simulink model "DAQ"  (R2014a)
settings: Solver=FixedStepDiscrete  StartTime=0.0  StopTime=inf  FixedStep=sample_time  RelTol=1e-3
values from neighbouring files (symbols this model uses):
  A_lpf_velocity = 1 + B1_lpf_velocity + B2_lpf_velocity    [daq_params.m]
  B1_lpf_velocity = -2*exp(-lpf_damping*fcut_velocity*sample_time)*cos(fcut_velocity*sample_time*sqrt(1-lpf_damping^2))    [daq_params.m]
  B2_lpf_velocity = exp(-2*lpf_damping*fcut_velocity*sample_time)    [daq_params.m]
  BOOM_MAX_ENCODER_TICKS = 2^17 - 1    (= 131071)    [daq_params.m]
  BOOM_PITCH_CAL_VALUE_RAD = 0    [daq_params.m]
  BOOM_PITCH_CAL_VALUE_TICKS = 63515    [daq_params.m]
  BOOM_PITCH_ENCODER_RAD_PER_TICK = 2*pi / (2^17 * 2)    (= 2.39684498107e-05)    [daq_params.m]
  BOOM_ROLL_CAL_VALUE_RAD = 6*pi/180    (= 0.10471975512)    [daq_params.m]
  BOOM_ROLL_CAL_VALUE_TICKS = 68304    [daq_params.m]
  BOOM_ROLL_ENCODER_RAD_PER_TICK = 2*pi / (2^17 * 7)    (= 6.84812851735e-06)    [daq_params.m]
  BOOM_YAW_ENCODER_RAD_PER_TICK = 2*pi / (2^17 * 9.6)    (= 4.9934270439e-06)    [daq_params.m]
  fcut_smooth = 16*(2*pi)    (= 100.530964915)    [daq_params.m]
  fcut_unwrap = 8*(2*pi)    (= 50.2654824574)    [daq_params.m]
  HIP_ABS_ENCODER_RAD_PER_TICK = 2*pi / 2^13    (= 0.000766990393943)    [daq_params.m]
  HIP_ABS_MAX_ENCODER_TICKS = 2^13 - 1    (= 8191)    [daq_params.m]
  HIP_INC_ENCODER_RAD_PER_TICK = 2*pi / (2500 * 4 * 57)    (= 1.10231321179e-05)    [daq_params.m]
  HIP_INC_MAX_ENCODER_TICKS = 2^16 - 1    (= 65535)    [daq_params.m]
  HIP_MOTOR_CONSTANT = 0.184    [daq_params.m]
  HIP_MTR_GEAR_RATIO = 57    [daq_params.m]
  HIP_MTR_MAX_TORQUE = MTR_HIP_MAX_CURRENT*HIP_MOTOR_CONSTANT*HIP_MTR_GEAR_RATIO    (= 629.28)    [daq_params.m]
  LEFT_HIP_CALIB_POS = 3*pi/2    (= 4.71238898038)    [daq_params.m]
  LEFT_HIP_CALIB_VAL = 1359    [daq_params.m]
  LEFT_MOTOR_HIP_DIRECTION = 1.0    (= 1)    [daq_params.m]
  LEG1_LEG_A_CALIB_VAL = 227806296+18240-105494    (= 227719042)    [daq_params.m]
  LEG1_LEG_A_RAD_PER_CNT = 9.8039216e-09    [daq_params.m]
  LEG1_LEG_B_CALIB_VAL = 227981518-27550+100498    (= 228054466)    [daq_params.m]
  LEG1_LEG_B_RAD_PER_CNT = -9.8039216e-09    [daq_params.m]
  LEG1_MOTOR_A_DIRECTION = 1.0    (= 1)    [daq_params.m]
  LEG1_MOTOR_B_DIRECTION = -1.0    (= -1)    [daq_params.m]
  LEG1_TRAN_A_CALIB_VAL = 162551054    [daq_params.m]
  LEG1_TRAN_A_RAD_PER_CNT = 9.8039216e-09    [daq_params.m]
  LEG1_TRAN_B_CALIB_VAL = 163658926    [daq_params.m]
  LEG1_TRAN_B_RAD_PER_CNT = -9.8039216e-09    [daq_params.m]
  LEG2_LEG_A_CALIB_VAL = 208914429-56335+74466    (= 208932560)    [daq_params.m]
  LEG2_LEG_A_RAD_PER_CNT = -9.8039216e-09    [daq_params.m]
  LEG2_LEG_B_CALIB_VAL = 229010442-9300+102681    (= 229103823)    [daq_params.m]
  LEG2_LEG_B_RAD_PER_CNT = -9.8039216e-09    [daq_params.m]
  LEG2_MOTOR_A_DIRECTION = 1.0    (= 1)    [daq_params.m]
  LEG2_MOTOR_B_DIRECTION = -1.0    (= -1)    [daq_params.m]
  LEG2_TRAN_A_CALIB_VAL = 162423925    [daq_params.m]
  LEG2_TRAN_A_RAD_PER_CNT = 9.8039216e-09    [daq_params.m]
  LEG2_TRAN_B_CALIB_VAL = 177684487    [daq_params.m]
  LEG2_TRAN_B_RAD_PER_CNT = 9.8039216e-09    [daq_params.m]
  LEG_A_CALIB_LOC = 0.959931088596881    (= 0.959931088597)    [daq_params.m]
  LEG_B_CALIB_LOC = 2.181661564992912    (= 2.18166156499)    [daq_params.m]
  LEG_MOTOR_CONSTANT = 0.119    [daq_params.m]
  LEG_MTR_GEAR_RATIO = 50    [daq_params.m]
  LEG_MTR_MAX_TORQUE = MTR_MAX_CURRENT*LEG_MOTOR_CONSTANT*LEG_MTR_GEAR_RATIO    (= 357)    [daq_params.m]
  max_encoder_velocity = 200    [daq_params.m]
  MTR_HIP_MAX_CURRENT = 60.0    (= 60)    [daq_params.m]
  MTR_MAX_COUNT = 19900    [daq_params.m]
  MTR_MAX_CURRENT = 60.0    (= 60)    [daq_params.m]
  RIGHT_HIP_CALIB_POS = -pi/2    (= -1.57079632679)    [daq_params.m]
  RIGHT_HIP_CALIB_VAL = 4444    [daq_params.m]
  RIGHT_MOTOR_HIP_DIRECTION = 1.0    (= 1)    [daq_params.m]
  sensor_start_time = 8    [daq_params.m]
undefined symbols (not defined in the file or in its folder): max_sensor_velocity, sample_time
libraries: xpcethercatlib x158, simulink x15, dspswit3 x1
(part 1 of 3)
settings Model: xpc_rtwmakecfg_data=_xpcethercatlib_  BufferReuse=off  Creator=wmartin  LastModifiedBy=wmartin
settings SolverCC: EnableConcurrentExecution=on
settings DataIOCC: MaxDataPoints=1000000000  SaveFormat=StructureWithTime  SaveOutput=off  SaveTime=off
settings OptimizationCC: BlockReduction=off  OptimizeBlockIOStorage=off  BufferReuse=off  GlobalBufferReuse=off  ExpressionFolding=off  ExpressionDepthLimit=2147483647  LocalBlockOutputs=off  SimCompilerOptimization=On
settings DebuggingCC: UnderspecifiedInitializationDetection=Classic  StateNameClashWarn=warning
settings HardwareCC: ProdIntDivRoundTo=Zero  ProdEndianess=LittleEndian  ProdHWDeviceType=Generic->32-bit x86 compatible
settings ModelReferenceCC: ModelReferenceNumInstancesAllowed=Single  ModelReferenceMinAlgLoopOccurrences=on
settings RTWCC: SystemTargetFile=slrt.tlc  TemplateMakefile=slrt_default_tmf  Description=Simulink Real-Time  RTWVerbose=off  ProcessScript=slrt_make_rtw_hook  RTWCompilerOptimization=On
settings SimulinkRealTimeCC: GeneratePreprocessorConditionals=Disable all  EnableShiftOperators=on  RL32LogBufSizeModifier=100000000

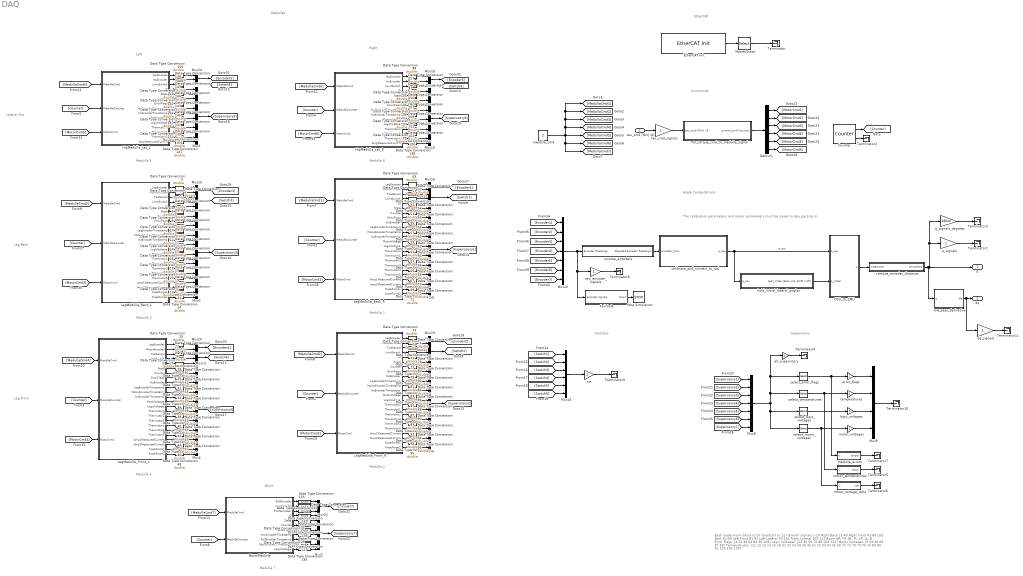
== system DAQ ==
  note: Left
  note: The calibration parameters and motor parameters
      | must be saved in daq_params.m
  note: Right
  note: Lateral Hip
  note: Leg Back
  note: Leg Front
  note: Boom
  note: Medullas
  note: EtherCAT
  note: Angle Computations
  note: Commands
  note: Switches
  note: Supervisory
  note: Medulla 1
  note: Medulla 2
  note: Medulla 4
  note: Medulla 3
  note: Medulla 5
  note: Medulla 6
  note: Medulla 7
  note: Each Supervisory block is 20 (sagittal) or 12 (lateral) signals
      | 1-20      Right Back
      | 21-40     Right Front
      | 41-60     Left Back
      | 61-80     Left Front
      | 81-92     Left Lateral
      | 93-104    Right Lateral
      | 105-112   Boom
      |
      | BR, FR, BL, FL, LR, LL, B
      | Error Flags: [4 24 44 64 84 96 108]
      | Logic Voltages: [10 30 50 70 88 100 112]
      | Motor Voltages: [9 29 49 69 87 99]
      | Temperatures: [11 12 13 14 15 16 31 32 33 34 35 36 51 52 53 54 55 56 71 72 73 74 75 76 89 90 91 101 102 103]
  tau_cmd [Nm] x6 : Inport  OutDataTypeStr=double  PortDimensions=6  SampleTime=0
  BoomMedulla : Subsystem
  Counter : dspswit3/Counter  Direction=Up  CountEvent=Free running  CounterSize=User defined  MaxCount=65535  InitialCount=0  Output=Count and Hit  HitValue=32  ResetInput=off  SamplesPerFrame=1  Ts=.001  CntDtype=double  HitDtype=Logical
  Data Type Conversion{1..111,127..151,157} (137 alike) : DataTypeConversion  OutDataTypeStr=double
  Demux1 : Demux  Outputs=6
  EtherCAT Init : xpcethercatlib/EtherCAT Init   Priority=0  config_file=C:\Users\wmartin\Dropbox\research\atrias\atrias-controller\00 Global Files\atrias_boom.xml  device_id=0  pci_bus=2  pci_slot=2  enaDebug=off  enaDC=on  errLink=off  masterDbg=off  stateChgDbg=off  baseClock=off  masterCfg=off  logFile='E:\dbglog.txt'  sample_time=0.001000
  Fail Safe : Subsystem
  HipMedulla_Lat_L : Subsystem
  HipMedulla_Lat_R : Subsystem
  LegMedulla_Back_L : Subsystem
  LegMedulla_Back_R : Subsystem
  LegMedulla_Front_L : Subsystem
  LegMedulla_Front_R : Subsystem
  MasterState : Selector  InputPortWidth=6  Indices=[2]
  Mux1 : Mux  Inputs=12
  Mux10 : Mux  Inputs=12
  Mux{2,11..13,15..16,18..20,24} (10 alike) : Mux  Inputs=2
  Mux14 : Mux  Inputs=6
  Mux21 : Mux  Inputs=3
  Mux22 : Mux  Inputs=7
  Mux{3..6} (4 alike) : Mux  Inputs=20
  Mux7 : Mux  Inputs=8
  Mux8 : Mux  Inputs=7
  Mux9 : Mux
  OSU_to_CMU : Subsystem
  Stop Simulation : Stop
  Terminator{,1..11} (12 alike) : Terminator
  all_supervisory : Gain
  calibrate_and_convert_to_rad : Subsystem
  dq_signals : Gain
  error_flags : Gain
  hold_initial_lateral_angles : Subsystem
  logic_voltages : Gain
  low_pass_derivative : Subsystem
  medulla_cmd : Constant  Value=2
  medulla_errors : MATLAB Function  TreatAsAtomicUnit=on
  motor_temperatures : MATLAB Function  TreatAsAtomicUnit=on
  motor_voltage_volts : MATLAB Function  TreatAsAtomicUnit=on
  motor_voltages : Gain
  mtr_torque_cmd_to_medulla_signal : Subsystem
  q_signals : Gain
  q_signals_degrees : Gain  Gain=180/pi
  raw_encoder_signals : Gain
  remove_encoder_dropouts : Subsystem
  select_error_flags : Selector  InputPortWidth=112  Indices=[4 24 44 64 84 96 108]
  select_logic_voltages : Selector  InputPortWidth=112  Indices=[10 30 50 70 88 100 112]
  select_motor_voltages : Selector  InputPortWidth=112  Indices=[9 29 49 69 87 99]
  select_temperatures : Selector  InputPortWidth=112  Indices=[11 12 13 14 15 16 31 32 33 34 35 36 51 52 53 54 55 56 71 72 73 74 75 76 89 90 91 101 102 103]
  sw : Gain
  tau_cmd_signals : Gain
  temperatures : Gain
  unwrap_encoders : Subsystem
  q : Outport  OutDataTypeStr=double  PortDimensions=13  SampleTime=[0.001,0]
  dq : Outport  Port=2  OutDataTypeStr=double  PortDimensions=13  SampleTime=[0.001,0]
  wires:
  BoomMedulla/11(LogicVoltage) -> Data Type Conversion136/1
  BoomMedulla/10(PitchEncoderTimestamp) -> Data Type Conversion137/1
  BoomMedulla/9(RollEncoderTimestamp) -> Data Type Conversion127/1
  BoomMedulla/8(YawEncoderTimestamp) -> Data Type Conversion129/1
  BoomMedulla/7(ErrorFlags) -> Data Type Conversion130/1
  BoomMedulla/6(Counter) -> Data Type Conversion128/1
  BoomMedulla/5(State) -> Data Type Conversion134/1
  BoomMedulla/4(ID) -> Data Type Conversion135/1
  BoomMedulla/3(PitchEncoder) -> Data Type Conversion131/1
  BoomMedulla/2(YawEncoder) -> Data Type Conversion132/1
  BoomMedulla/1(RollEncoder) -> Data Type Conversion133/1
  Data Type Conversion133/1 -> Mux21/1
  Data Type Conversion132/1 -> Mux21/2
  Data Type Conversion131/1 -> Mux21/3
  Data Type Conversion135/1 -> Mux7/1
  Data Type Conversion134/1 -> Mux7/2
  Data Type Conversion128/1 -> Mux7/3
  Data Type Conversion130/1 -> Mux7/4
  Data Type Conversion129/1 -> Mux7/5
  Data Type Conversion127/1 -> Mux7/6
  Data Type Conversion137/1 -> Mux7/7
  Data Type Conversion136/1 -> Mux7/8
  HipMedulla_Lat_R/15(AmpMeasuredCurrent) -> Data Type Conversion138/1
  HipMedulla_Lat_R/14(Thermistor2) -> Data Type Conversion99/1
  HipMedulla_Lat_R/13(Thermistor1) -> Data Type Conversion100/1
  HipMedulla_Lat_R/12(Thermistor0) -> Data Type Conversion102/1
  HipMedulla_Lat_R/11(LogicVoltage) -> Data Type Conversion103/1
  HipMedulla_Lat_R/10(MotorVoltage) -> Data Type Conversion101/1
  HipMedulla_Lat_R/9(IncEncoderTimestamp) -> Data Type Conversion108/1
  HipMedulla_Lat_R/8(HipEncoderTimestamp) -> Data Type Conversion109/1
  HipMedulla_Lat_R/7(ErrorFlags) -> Data Type Conversion106/1
  HipMedulla_Lat_R/6(Counter) -> Data Type Conversion107/1
  HipMedulla_Lat_R/5(State) -> Data Type Conversion105/1
  HipMedulla_Lat_R/4(ID) -> Data Type Conversion110/1
  HipMedulla_Lat_R/3(LimitSwitch) -> Data Type Conversion157/1
  HipMedulla_Lat_R/2(IncEncoder) -> Data Type Conversion97/1
  HipMedulla_Lat_R/1(HipEncoder) -> Data Type Conversion98/1
  Data Type Conversion98/1 -> Mux18/1
  Data Type Conversion97/1 -> Mux18/2
  Data Type Conversion110/1 -> Mux10/1
  Data Type Conversion105/1 -> Mux10/2
  Data Type Conversion107/1 -> Mux10/3
  Data Type Conversion106/1 -> Mux10/4
  Data Type Conversion109/1 -> Mux10/5
  Data Type Conversion108/1 -> Mux10/6
  Data Type Conversion101/1 -> Mux10/7
  Data Type Conversion103/1 -> Mux10/8
  Data Type Conversion102/1 -> Mux10/9
  Data Type Conversion100/1 -> Mux10/10
  Data Type Conversion99/1 -> Mux10/11
  mtr_torque_cmd_to_medulla_signal/1(current_cmd [counts]) -> Demux1/1
  Data Type Conversion50/1 -> Mux16/2
  Data Type Conversion49/1 -> Mux16/1
  Data Type Conversion48/1 -> Mux4/20
  Data Type Conversion47/1 -> Mux4/19
  Data Type Conversion46/1 -> Mux4/18
  Data Type Conversion45/1 -> Mux4/17
  Data Type Conversion44/1 -> Mux4/16
  Data Type Conversion43/1 -> Mux4/15
  Data Type Conversion42/1 -> Mux4/14
  Data Type Conversion41/1 -> Mux4/13
  Data Type Conversion40/1 -> Mux4/12
  Data Type Conversion39/1 -> Mux4/11
  Data Type Conversion38/1 -> Mux4/10
  Data Type Conversion37/1 -> Mux4/9
  Data Type Conversion36/1 -> Mux4/8
  Data Type Conversion35/1 -> Mux4/7
  Data Type Conversion34/1 -> Mux4/6
  Data Type Conversion33/1 -> Mux4/5
  Data Type Conversion32/1 -> Mux4/4
  Data Type Conversion31/1 -> Mux4/3
  Data Type Conversion30/1 -> Mux4/2
  Data Type Conversion29/1 -> Mux4/1
  Data Type Conversion28/1 -> Mux13/2
  Data Type Conversion27/1 -> Mux13/1
  Data Type Conversion26/1 -> Mux20/2
  Data Type Conversion25/1 -> Mux20/1
  Data Type Conversion24/1 -> Mux3/20
  Data Type Conversion23/1 -> Mux3/19
  Data Type Conversion22/1 -> Mux3/18
  Data Type Conversion21/1 -> Mux3/17
  Data Type Conversion20/1 -> Mux3/16
  Data Type Conversion19/1 -> Mux3/15
  Data Type Conversion18/1 -> Mux3/14
  Data Type Conversion17/1 -> Mux3/13
  Data Type Conversion16/1 -> Mux3/12
  Data Type Conversion15/1 -> Mux3/11
  Data Type Conversion14/1 -> Mux3/10
  Data Type Conversion13/1 -> Mux3/9
  Data Type Conversion12/1 -> Mux3/8
  Data Type Conversion11/1 -> Mux3/7
  Data Type Conversion10/1 -> Mux3/6
  Data Type Conversion9/1 -> Mux3/5
  Data Type Conversion8/1 -> Mux3/4
  Data Type Conversion7/1 -> Mux3/3
  Data Type Conversion6/1 -> Mux3/2
  Data Type Conversion5/1 -> Mux3/1
  Data Type Conversion4/1 -> Mux2/2
  Data Type Conversion2/1 -> Mux2/1
  Data Type Conversion1/1 -> Mux15/2
  Data Type Conversion3/1 -> Mux15/1
  LegMedulla_Back_R/1(LegEncoder) -> Data Type Conversion49/1
  LegMedulla_Back_L/1(LegEncoder) -> Data Type Conversion3/1
  LegMedulla_Back_R/2(MotorEncoder) -> Data Type Conversion50/1
  tau_cmd [Nm] x6/1 -> tau_cmd_signals/1
  Data Type Conversion138/1 -> Mux10/12
  Data Type Conversion96/1 -> Mux6/20
  Data Type Conversion95/1 -> Mux6/19
  Data Type Conversion94/1 -> Mux6/18
  Data Type Conversion93/1 -> Mux6/17
  Data Type Conversion92/1 -> Mux6/16
  Data Type Conversion91/1 -> Mux6/15
  Data Type Conversion90/1 -> Mux6/14
  Data Type Conversion89/1 -> Mux6/13
  Data Type Conversion88/1 -> Mux6/12
  Data Type Conversion87/1 -> Mux6/11
  Data Type Conversion86/1 -> Mux6/10
  Data Type Conversion85/1 -> Mux6/9
  Data Type Conversion84/1 -> Mux6/8
  Data Type Conversion83/1 -> Mux6/7
  Data Type Conversion82/1 -> Mux6/6
  Data Type Conversion81/1 -> Mux6/5
  Data Type Conversion80/1 -> Mux6/4
  Data Type Conversion79/1 -> Mux6/3
  Data Type Conversion78/1 -> Mux6/2
  Data Type Conversion77/1 -> Mux6/1
  Data Type Conversion76/1 -> Mux12/2
  Data Type Conversion75/1 -> Mux12/1
  Data Type Conversion74/1 -> Mux19/2
  Data Type Conversion73/1 -> Mux19/1
  Data Type Conversion72/1 -> Mux5/20
  Data Type Conversion71/1 -> Mux5/19
  Data Type Conversion70/1 -> Mux5/18
  Data Type Conversion69/1 -> Mux5/17
  Data Type Conversion68/1 -> Mux5/16
  Data Type Conversion67/1 -> Mux5/15
  Data Type Conversion66/1 -> Mux5/14
  Data Type Conversion65/1 -> Mux5/13
  Data Type Conversion64/1 -> Mux5/12
  Data Type Conversion63/1 -> Mux5/11
  Data Type Conversion62/1 -> Mux5/10
  Data Type Conversion61/1 -> Mux5/9
  Data Type Conversion60/1 -> Mux5/8
  Data Type Conversion59/1 -> Mux5/7
  Data Type Conversion58/1 -> Mux5/6
  Data Type Conversion57/1 -> Mux5/5
  Data Type Conversion56/1 -> Mux5/4
  Data Type Conversion55/1 -> Mux5/3
  Data Type Conversion54/1 -> Mux5/2
  Data Type Conversion53/1 -> Mux5/1
  Data Type Conversion52/1 -> Mux11/2
  Data Type Conversion51/1 -> Mux11/1
  LegMedulla_Front_R/3(ToeSensor) -> Data Type Conversion75/1
  LegMedulla_Front_R/2(MotorEncoder) -> Data Type Conversion74/1
  LegMedulla_Front_R/1(LegEncoder) -> Data Type Conversion73/1
  Counter/2 -> Terminator2/1
  LegMedulla_Front_R/24(KneeForce2) -> Data Type Conversion96/1
  LegMedulla_Back_R/24(KneeForce2) -> Data Type Conversion72/1
  LegMedulla_Front_R/23(KneeForce1) -> Data Type Conversion95/1
  LegMedulla_Front_R/22(Amp2MeasuredCurrent) -> Data Type Conversion94/1
  LegMedulla_Front_R/21(Amp1MeasuredCurrent) -> Data Type Conversion93/1
  LegMedulla_Front_R/20(Thermistor5) -> Data Type Conversion92/1
  LegMedulla_Front_R/19(Thermistor4) -> Data Type Conversion91/1
  LegMedulla_Front_R/18(Thermistor3) -> Data Type Conversion90/1
  LegMedulla_Front_R/17(Thermistor2) -> Data Type Conversion89/1
  LegMedulla_Front_R/16(Thermistor1) -> Data Type Conversion88/1
  LegMedulla_Front_R/15(Thermistor0) -> Data Type Conversion87/1
  LegMedulla_Front_R/14(LogicVoltage) -> Data Type Conversion86/1
  LegMedulla_Front_R/13(MotorVoltage) -> Data Type Conversion85/1
  LegMedulla_Front_R/12(IncEncoderTimestamp) -> Data Type Conversion84/1
  LegMedulla_Front_R/11(MotorEncoderTimestamp) -> Data Type Conversion83/1
  LegMedulla_Front_R/10(LegEncoderTimestamp) -> Data Type Conversion82/1
  LegMedulla_Front_R/9(IncEncoder) -> Data Type Conversion81/1
  LegMedulla_Front_R/8(ErrorFlags) -> Data Type Conversion80/1
  LegMedulla_Front_R/7(Counter) -> Data Type Conversion79/1
  LegMedulla_Front_R/6(State) -> Data Type Conversion78/1
  LegMedulla_Front_R/5(ID) -> Data Type Conversion77/1
  LegMedulla_Front_R/4(LimitSwitch) -> Data Type Conversion76/1
  LegMedulla_Back_R/23(KneeForce1) -> Data Type Conversion71/1
  LegMedulla_Back_R/22(Amp2MeasuredCurrent) -> Data Type Conversion70/1
  LegMedulla_Back_R/21(Amp1MeasuredCurrent) -> Data Type Conversion69/1
  LegMedulla_Back_R/20(Thermistor5) -> Data Type Conversion68/1
  LegMedulla_Back_R/19(Thermistor4) -> Data Type Conversion67/1
  LegMedulla_Back_R/18(Thermistor3) -> Data Type Conversion66/1
  LegMedulla_Back_R/17(Thermistor2) -> Data Type Conversion65/1
  LegMedulla_Back_R/16(Thermistor1) -> Data Type Conversion64/1
  LegMedulla_Back_R/15(Thermistor0) -> Data Type Conversion63/1
  LegMedulla_Back_R/14(LogicVoltage) -> Data Type Conversion62/1
  LegMedulla_Back_R/13(MotorVoltage) -> Data Type Conversion61/1
  LegMedulla_Back_R/12(IncEncoderTimestamp) -> Data Type Conversion60/1
  LegMedulla_Back_R/11(MotorEncoderTimestamp) -> Data Type Conversion59/1
  LegMedulla_Back_R/10(LegEncoderTimestamp) -> Data Type Conversion58/1
  LegMedulla_Back_R/9(IncEncoder) -> Data Type Conversion57/1
  LegMedulla_Back_R/8(ErrorFlags) -> Data Type Conversion56/1
  LegMedulla_Back_R/7(Counter) -> Data Type Conversion55/1
  LegMedulla_Back_R/6(State) -> Data Type Conversion54/1
  LegMedulla_Back_R/5(ID) -> Data Type Conversion53/1
  LegMedulla_Back_R/4(LimitSwitch) -> Data Type Conversion52/1
  LegMedulla_Back_R/3(ToeSensor) -> Data Type Conversion51/1
  LegMedulla_Front_L/24(KneeForce2) -> Data Type Conversion48/1
  LegMedulla_Back_L/24(KneeForce2) -> Data Type Conversion24/1
  LegMedulla_Front_L/23(KneeForce1) -> Data Type Conversion47/1
  LegMedulla_Front_L/22(Amp2MeasuredCurrent) -> Data Type Conversion46/1
  LegMedulla_Front_L/21(Amp1MeasuredCurrent) -> Data Type Conversion45/1
  LegMedulla_Front_L/20(Thermistor5) -> Data Type Conversion44/1
  LegMedulla_Front_L/19(Thermistor4) -> Data Type Conversion43/1
  LegMedulla_Front_L/18(Thermistor3) -> Data Type Conversion42/1
  LegMedulla_Front_L/17(Thermistor2) -> Data Type Conversion41/1
  LegMedulla_Front_L/16(Thermistor1) -> Data Type Conversion40/1
  LegMedulla_Front_L/15(Thermistor0) -> Data Type Conversion39/1
  LegMedulla_Front_L/14(LogicVoltage) -> Data Type Conversion38/1
  LegMedulla_Front_L/13(MotorVoltage) -> Data Type Conversion37/1
  LegMedulla_Front_L/12(IncEncoderTimestamp) -> Data Type Conversion36/1
  LegMedulla_Front_L/11(MotorEncoderTimestamp) -> Data Type Conversion35/1
  LegMedulla_Front_L/10(LegEncoderTimestamp) -> Data Type Conversion34/1
  LegMedulla_Front_L/9(IncEncoder) -> Data Type Conversion33/1
  LegMedulla_Front_L/8(ErrorFlags) -> Data Type Conversion32/1
  LegMedulla_Front_L/7(Counter) -> Data Type Conversion31/1
  LegMedulla_Front_L/6(State) -> Data Type Conversion30/1
  LegMedulla_Front_L/5(ID) -> Data Type Conversion29/1
  LegMedulla_Front_L/4(LimitSwitch) -> Data Type Conversion28/1
  LegMedulla_Front_L/3(ToeSensor) -> Data Type Conversion27/1
  LegMedulla_Front_L/2(MotorEncoder) -> Data Type Conversion26/1
  LegMedulla_Front_L/1(LegEncoder) -> Data Type Conversion25/1
  LegMedulla_Back_L/23(KneeForce1) -> Data Type Conversion23/1
  LegMedulla_Back_L/22(Amp2MeasuredCurrent) -> Data Type Conversion22/1
  LegMedulla_Back_L/21(Amp1MeasuredCurrent) -> Data Type Conversion21/1
  LegMedulla_Back_L/20(Thermistor5) -> Data Type Conversion20/1
  LegMedulla_Back_L/19(Thermistor4) -> Data Type Conversion19/1
  LegMedulla_Back_L/18(Thermistor3) -> Data Type Conversion18/1
  LegMedulla_Back_L/17(Thermistor2) -> Data Type Conversion17/1
  LegMedulla_Back_L/16(Thermistor1) -> Data Type Conversion16/1
  LegMedulla_Back_L/15(Thermistor0) -> Data Type Conversion15/1
  LegMedulla_Back_L/14(LogicVoltage) -> Data Type Conversion14/1
  LegMedulla_Back_L/13(MotorVoltage) -> Data Type Conversion13/1
  LegMedulla_Back_L/12(IncEncoderTimestamp) -> Data Type Conversion12/1
  LegMedulla_Back_L/11(MotorEncoderTimestamp) -> Data Type Conversion11/1
  LegMedulla_Back_L/10(LegEncoderTimestamp) -> Data Type Conversion10/1
  LegMedulla_Back_L/9(IncEncoder) -> Data Type Conversion9/1
  LegMedulla_Back_L/8(ErrorFlags) -> Data Type Conversion8/1
  LegMedulla_Back_L/7(Counter) -> Data Type Conversion7/1
  LegMedulla_Back_L/6(State) -> Data Type Conversion6/1
  LegMedulla_Back_L/5(ID) -> Data Type Conversion5/1
  LegMedulla_Back_L/4(LimitSwitch) -> Data Type Conversion4/1
  LegMedulla_Back_L/3(ToeSensor) -> Data Type Conversion2/1
  LegMedulla_Back_L/2(MotorEncoder) -> Data Type Conversion1/1
  Counter/1 -> [Counter]
  [Counter] -> LegMedulla_Back_L/2(MedullaCounter)
  [Counter] -> LegMedulla_Front_L/2(MedullaCounter)
  [Counter] -> LegMedulla_Back_R/2(MedullaCounter)
  [Counter] -> LegMedulla_Front_R/2(MedullaCounter)
  [Counter] -> HipMedulla_Lat_R/2(MedullaCounter)
  [Counter] -> HipMedulla_Lat_L/2(MedullaCounter)
  [Counter] -> BoomMedulla/2(MedullaCounter)
  medulla_cmd/1 -> [MedullaCmd7], [MedullaCmd6], [MedullaCmd5], [MedullaCmd4], [MedullaCmd3], [MedullaCmd2], [MedullaCmd1]
  [MedullaCmd3] -> LegMedulla_Back_L/1(MedullaCmd)
  [MedullaCmd4] -> LegMedulla_Front_L/1(MedullaCmd)
  [MedullaCmd1] -> LegMedulla_Back_R/1(MedullaCmd)
  [MedullaCmd2] -> LegMedulla_Front_R/1(MedullaCmd)
  [MedullaCmd6] -> HipMedulla_Lat_R/1(MedullaCmd)
  [MedullaCmd7] -> BoomMedulla/1(MedullaCmd)
  [MedullaCmd5] -> HipMedulla_Lat_L/1(MedullaCmd)
  Data Type Conversion157/1 -> [Switch6]
  [Switch1] -> Mux14/1
  [Switch2] -> Mux14/2
  [Switch3] -> Mux14/3
  [Switch4] -> Mux14/4
  [Switch5] -> Mux14/5
  [Switch6] -> Mux14/6
  low_pass_derivative/1(dq) -> dq_signals/1, dq/1
  calibrate_and_convert_to_rad/1(q_osu) -> OSU_to_CMU/1(q_osu), hold_initial_lateral_angles/1(q_osu)  "q_osu"
  hold_initial_lateral_angles/1(qLat_initial [absL incL absR incR]) -> OSU_to_CMU/2(q_initial)
  [MotorCmd3] -> LegMedulla_Back_L/3(MotorCmd)
  [MotorCmd4] -> LegMedulla_Front_L/3(MotorCmd)
  [MotorCmd1] -> LegMedulla_Back_R/3(MotorCmd)
  [MotorCmd2] -> LegMedulla_Front_R/3(MotorCmd)
  [MotorCmd6] -> HipMedulla_Lat_R/3(MotorCmd)
  [MotorCmd5] -> HipMedulla_Lat_L/3(MotorCmd)
  Demux1/1 -> [MotorCmd1]
  Demux1/2 -> [MotorCmd2]
  Demux1/3 -> [MotorCmd3]
  Demux1/4 -> [MotorCmd4]
  Demux1/5 -> [MotorCmd5]
  Demux1/6 -> [MotorCmd6]
  Mux2/1 -> [Switch3]
  Mux3/1 -> [Supervisory3]
  Mux4/1 -> [Supervisory4]
  Mux5/1 -> [Supervisory1]
  Mux6/1 -> [Supervisory2]
  Mux7/1 -> [Supervisory7]
  [Supervisory1] -> Mux8/1
  [Supervisory2] -> Mux8/2
  [Supervisory3] -> Mux8/3
  [Supervisory4] -> Mux8/4
  [Supervisory5] -> Mux8/5
  [Supervisory6] -> Mux8/6
  [Supervisory7] -> Mux8/7
  Mux10/1 -> [Supervisory6]
  Mux11/1 -> [Switch1]
  Mux12/1 -> [Switch2]
  Mux13/1 -> [Switch4]
  Mux14/1 -> sw/1
  Mux15/1 -> [Encoder3]
  Mux16/1 -> [Encoder1]
  Mux18/1 -> [Encoder6]
  Mux19/1 -> [Encoder2]
  Mux20/1 -> [Encoder4]
  Mux21/1 -> [Encoder7]
  [Encoder7] -> Mux22/7
  [Encoder6] -> Mux22/6
  [Encoder5] -> Mux22/5
  [Encoder4] -> Mux22/4
  [Encoder3] -> Mux22/3
  [Encoder2] -> Mux22/2
  [Encoder1] -> Mux22/1
  Mux22/1 -> unwrap_encoders/1(Encoder Readings), raw_encoder_signals/1, Fail Safe/1(encoder signals)
  HipMedulla_Lat_L/15(AmpMeasuredCurrent) -> Data Type Conversion147/1
  HipMedulla_Lat_L/14(Thermistor2) -> Data Type Conversion151/1
  HipMedulla_Lat_L/13(Thermistor1) -> Data Type Conversion104/1
  HipMedulla_Lat_L/12(Thermistor0) -> Data Type Conversion139/1
  HipMedulla_Lat_L/11(LogicVoltage) -> Data Type Conversion140/1
  HipMedulla_Lat_L/10(MotorVoltage) -> Data Type Conversion111/1
  HipMedulla_Lat_L/9(IncEncoderTimestamp) -> Data Type Conversion144/1
  HipMedulla_Lat_L/8(HipEncoderTimestamp) -> Data Type Conversion145/1
  HipMedulla_Lat_L/7(ErrorFlags) -> Data Type Conversion142/1
  HipMedulla_Lat_L/6(Counter) -> Data Type Conversion143/1
  HipMedulla_Lat_L/5(State) -> Data Type Conversion141/1
  HipMedulla_Lat_L/4(ID) -> Data Type Conversion146/1
  HipMedulla_Lat_L/3(LimitSwitch) -> Data Type Conversion148/1
  HipMedulla_Lat_L/2(IncEncoder) -> Data Type Conversion149/1
  HipMedulla_Lat_L/1(HipEncoder) -> Data Type Conversion150/1
  Data Type Conversion150/1 -> Mux24/1
  Data Type Conversion149/1 -> Mux24/2
  Data Type Conversion146/1 -> Mux1/1
  Data Type Conversion141/1 -> Mux1/2
  Data Type Conversion143/1 -> Mux1/3
  Data Type Conversion142/1 -> Mux1/4
  Data Type Conversion145/1 -> Mux1/5
  Data Type Conversion144/1 -> Mux1/6
  Data Type Conversion111/1 -> Mux1/7
  Data Type Conversion140/1 -> Mux1/8
  Data Type Conversion139/1 -> Mux1/9
  Data Type Conversion104/1 -> Mux1/10
  Data Type Conversion151/1 -> Mux1/11
  Data Type Conversion147/1 -> Mux1/12
  Data Type Conversion148/1 -> [Switch5]
  Mux1/1 -> [Supervisory5]
  Mux24/1 -> [Encoder5]
  q_signals/1 -> Terminator1/1
  tau_cmd_signals/1 -> mtr_torque_cmd_to_medulla_signal/1(tau_cmd [Nm] x6)
  Mux8/1 -> select_temperatures/1, select_error_flags/1, all_supervisory/1, select_motor_voltages/1, select_logic_voltages/1
  select_error_flags/1 -> error_flags/1, medulla_errors/1(u)
  select_temperatures/1 -> temperatures/1, motor_temperatures/1(u)
  select_logic_voltages/1 -> logic_voltages/1
  select_motor_voltages/1 -> motor_voltages/1, motor_voltage_volts/1(u)
  error_flags/1 -> Mux9/1
  temperatures/1 -> Mux9/2
  logic_voltages/1 -> Mux9/3
  motor_voltages/1 -> Mux9/4
  Mux9/1 -> Terminator10/1
  q_signals_degrees/1 -> Terminator3/1
  OSU_to_CMU/1(q) -> remove_encoder_dropouts/1(measured)
  EtherCAT Init/1 -> MasterState/1
  all_supervisory/1 -> Terminator4/1
  motor_temperatures/1(temp) -> Terminator5/1
  motor_voltage_volts/1(volt) -> Terminator6/1
  medulla_errors/1(errors) -> Terminator7/1
  MasterState/1 -> Terminator/1
  raw_encoder_signals/1 -> Terminator8/1
  sw/1 -> Terminator9/1
  remove_encoder_dropouts/1(smoothed) -> low_pass_derivative/1(q), q_signals/1, q_signals_degrees/1, q/1
  unwrap_encoders/1(Adjusted Encoder Readings) -> calibrate_and_convert_to_rad/1(encoder_ticks)
  Fail Safe/1(stop?) -> Stop Simulation/1
  dq_signals/1 -> Terminator11/1

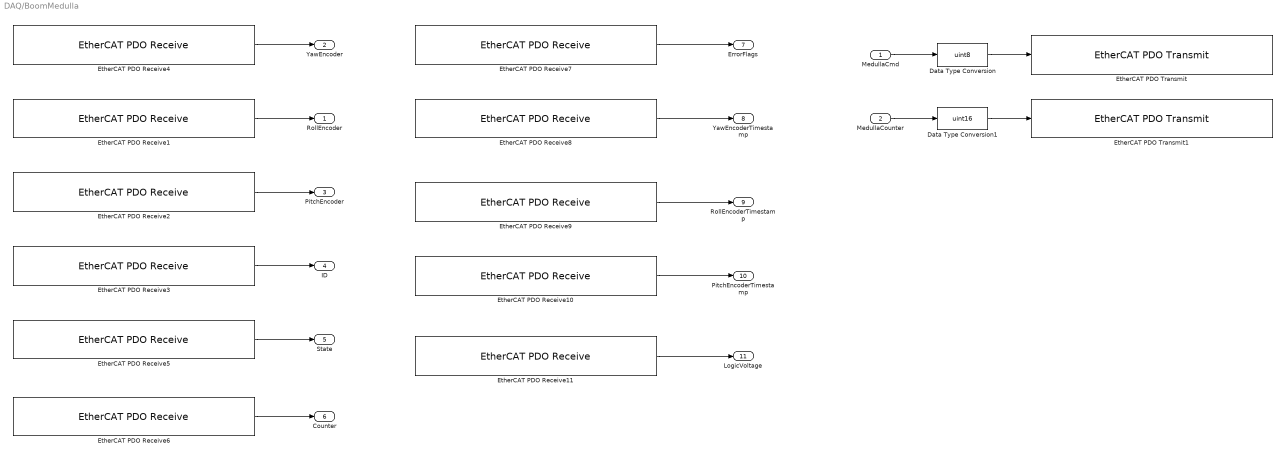
== system DAQ/BoomMedulla ==
  MedullaCmd : Inport
  MedullaCounter : Inport  Port=2
  Data Type Conversion : DataTypeConversion  OutDataTypeStr=uint8
  Data Type Conversion1 : DataTypeConversion  OutDataTypeStr=uint16
  EtherCAT PDO Receive1 : xpcethercatlib/EtherCAT PDO Receive  Priority=2  sig_name=Box 7 (ATRIAS 2.1 Boom (Medulla 1.5)).X Encoder.Encoder  sig_offset=2432  sig_type=uint32  type_size=32  sig_dim=1  device_id=0  sample_time=0.001000
  EtherCAT PDO Receive10 : xpcethercatlib/EtherCAT PDO Receive  Priority=2  sig_name=Box 7 (ATRIAS 2.1 Boom (Medulla 1.5)).Pitch Encoder.Timestamp  sig_offset=2512  sig_type=uint16  type_size=16  sig_dim=1  device_id=0  sample_time=0.001000
  EtherCAT PDO Receive11 : xpcethercatlib/EtherCAT PDO Receive  Priority=2  sig_name=Box 7 (ATRIAS 2.1 Boom (Medulla 1.5)).Power.Logic Voltage  sig_offset=2576  sig_type=uint16  type_size=16  sig_dim=1  device_id=0  sample_time=0.001000
  EtherCAT PDO Receive2 : xpcethercatlib/EtherCAT PDO Receive  Priority=2  sig_name=Box 7 (ATRIAS 2.1 Boom (Medulla 1.5)).Pitch Encoder.Encoder  sig_offset=2480  sig_type=uint32  type_size=32  sig_dim=1  device_id=0  sample_time=0.001000
  EtherCAT PDO Receive3 : xpcethercatlib/EtherCAT PDO Receive  Priority=2  sig_name=Box 7 (ATRIAS 2.1 Boom (Medulla 1.5)).uController Status.ID  sig_offset=2400  sig_type=uint8  type_size=8  sig_dim=1  device_id=0  sample_time=0.001000
  EtherCAT PDO Receive4 : xpcethercatlib/EtherCAT PDO Receive  Priority=2  sig_name=Box 7 (ATRIAS 2.1 Boom (Medulla 1.5)).Z Encoder.Encoder  sig_offset=2528  sig_type=uint32  type_size=32  sig_dim=1  device_id=0  sample_time=0.001000
  EtherCAT PDO Receive5 : xpcethercatlib/EtherCAT PDO Receive  Priority=2  sig_name=Box 7 (ATRIAS 2.1 Boom (Medulla 1.5)).uController Status.State  sig_offset=2408  sig_type=uint8  type_size=8  sig_dim=1  device_id=0  sample_time=0.001000
  EtherCAT PDO Receive6 : xpcethercatlib/EtherCAT PDO Receive  Priority=2  sig_name=Box 7 (ATRIAS 2.1 Boom (Medulla 1.5)).uController Status.Counter  sig_offset=2416  sig_type=uint8  type_size=8  sig_dim=1  device_id=0  sample_time=0.001000
  EtherCAT PDO Receive7 : xpcethercatlib/EtherCAT PDO Receive  Priority=2  sig_name=Box 7 (ATRIAS 2.1 Boom (Medulla 1.5)).uController Status.Error Flags  sig_offset=2424  sig_type=uint8  type_size=8  sig_dim=1  device_id=0  sample_time=0.001000
  EtherCAT PDO Receive8 : xpcethercatlib/EtherCAT PDO Receive  Priority=2  sig_name=Box 7 (ATRIAS 2.1 Boom (Medulla 1.5)).Z Encoder.Timestamp  sig_offset=2560  sig_type=uint16  type_size=16  sig_dim=1  device_id=0  sample_time=0.001000
  EtherCAT PDO Receive9 : xpcethercatlib/EtherCAT PDO Receive  Priority=2  sig_name=Box 7 (ATRIAS 2.1 Boom (Medulla 1.5)).X Encoder.Timestamp  sig_offset=2464  sig_type=uint16  type_size=16  sig_dim=1  device_id=0  sample_time=0.001000
  EtherCAT PDO Transmit : xpcethercatlib/EtherCAT PDO Transmit   Priority=3  sig_name=Box 7 (ATRIAS 2.1 Boom (Medulla 1.5)).uControllerInput.Command  sig_offset=2400  sig_type=uint8  type_size=8  sig_dim=1  device_id=0  sample_time=0.001000
  EtherCAT PDO Transmit1 : xpcethercatlib/EtherCAT PDO Transmit   Priority=3  sig_name=Box 7 (ATRIAS 2.1 Boom (Medulla 1.5)).uControllerInput.Counter  sig_offset=2408  sig_type=uint16  type_size=16  sig_dim=1  device_id=0  sample_time=0.001000
  RollEncoder : Outport
  YawEncoder : Outport  Port=2
  PitchEncoder : Outport  Port=3
  ID : Outport  Port=4
  State : Outport  Port=5
  Counter : Outport  Port=6
  ErrorFlags : Outport  Port=7
  YawEncoderTimestamp : Outport  Port=8
  RollEncoderTimestamp : Outport  Port=9
  PitchEncoderTimestamp : Outport  Port=10
  LogicVoltage : Outport  Port=11
  wires:
  Data Type Conversion/1 -> EtherCAT PDO Transmit/1
  Data Type Conversion1/1 -> EtherCAT PDO Transmit1/1
  MedullaCmd/1 -> Data Type Conversion/1
  MedullaCounter/1 -> Data Type Conversion1/1
  EtherCAT PDO Receive4/1 -> YawEncoder/1
  EtherCAT PDO Receive1/1 -> RollEncoder/1
  EtherCAT PDO Receive2/1 -> PitchEncoder/1
  EtherCAT PDO Receive3/1 -> ID/1
  EtherCAT PDO Receive5/1 -> State/1
  EtherCAT PDO Receive6/1 -> Counter/1
  EtherCAT PDO Receive7/1 -> ErrorFlags/1
  EtherCAT PDO Receive8/1 -> YawEncoderTimestamp/1
  EtherCAT PDO Receive9/1 -> RollEncoderTimestamp/1
  EtherCAT PDO Receive10/1 -> PitchEncoderTimestamp/1
  EtherCAT PDO Receive11/1 -> LogicVoltage/1

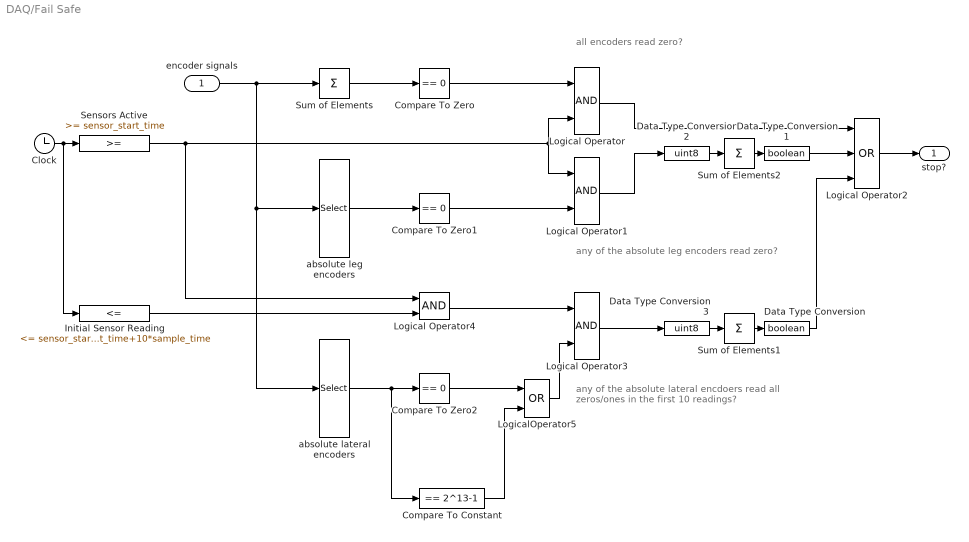
== system DAQ/Fail Safe ==
  note: any of the absolute leg encoders read zero?
  note: all encoders read zero?
  note: any of the absolute lateral encdoers read all
      | zeros/ones in the first 10 readings?
  encoder signals : Inport
  Clock : Clock
  Compare To Constant : simulink/Logic and Bit Operations/Compare To Constant  relop===  const=2^13-1  OutDataTypeStr=boolean
  Compare To Zero : simulink/Logic and Bit Operations/Compare To Zero  relop===  OutDataTypeStr=boolean
  Compare To Zero1 : simulink/Logic and Bit Operations/Compare To Zero  relop===  OutDataTypeStr=boolean
  Compare To Zero2 : simulink/Logic and Bit Operations/Compare To Zero  relop===  OutDataTypeStr=boolean
  Data Type Conversion : DataTypeConversion  OutDataTypeStr=boolean
  Data Type Conversion1 : DataTypeConversion  OutDataTypeStr=boolean
  Data Type Conversion2 : DataTypeConversion  OutDataTypeStr=uint8
  Data Type Conversion3 : DataTypeConversion  OutDataTypeStr=uint8
  Initial Sensor Reading : simulink/Logic and Bit Operations/Compare To Constant  relop=<=  const=sensor_start_time+10*sample_time  OutDataTypeStr=boolean
  Logical Operator{,1,3..4} (4 alike) : Logic  AllPortsSameDT=off  OutDataTypeStr=boolean
  Logical Operator2 : Logic  Operator=OR  Inputs=3  AllPortsSameDT=off  OutDataTypeStr=boolean
  LogicalOperator5 : Logic  Operator=OR  AllPortsSameDT=off  OutDataTypeStr=boolean
  Sensors Active : simulink/Logic and Bit Operations/Compare To Constant  relop=>=  const=sensor_start_time  OutDataTypeStr=boolean
  Sum of Elements : Sum  Inputs=+
  Sum of Elements1 : Sum  Inputs=+
  Sum of Elements2 : Sum  Inputs=+
  absolute lateral encoders : Selector  InputPortWidth=15  Indices=[9 11]
  absolute leg encoders : Selector  InputPortWidth=15  Indices=[1 2 3 4 5 6 7 8]
  stop? : Outport
  wires:
  LogicalOperator5/1 -> Logical Operator3/2
  Compare To Constant/1 -> LogicalOperator5/2
  Compare To Zero2/1 -> LogicalOperator5/1
  absolute leg encoders/1 -> Compare To Zero1/1
  Compare To Zero1/1 -> Logical Operator1/2
  Logical Operator2/1 -> stop?/1
  Logical Operator1/1 -> Data Type Conversion2/1
  Compare To Zero/1 -> Logical Operator/1
  encoder signals/1 -> absolute lateral encoders/1, absolute leg encoders/1, Sum of Elements/1
  Logical Operator/1 -> Logical Operator2/1
  Sum of Elements/1 -> Compare To Zero/1
  Sensors Active/1 -> Logical Operator4/1, Logical Operator/2, Logical Operator1/1
  absolute lateral encoders/1 -> Compare To Zero2/1, Compare To Constant/1
  Clock/1 -> Initial Sensor Reading/1, Sensors Active/1
  Initial Sensor Reading/1 -> Logical Operator4/2
  Logical Operator4/1 -> Logical Operator3/1
  Logical Operator3/1 -> Data Type Conversion3/1
  Sum of Elements1/1 -> Data Type Conversion/1
  Sum of Elements2/1 -> Data Type Conversion1/1
  Data Type Conversion/1 -> Logical Operator2/3
  Data Type Conversion1/1 -> Logical Operator2/2
  Data Type Conversion2/1 -> Sum of Elements2/1
  Data Type Conversion3/1 -> Sum of Elements1/1

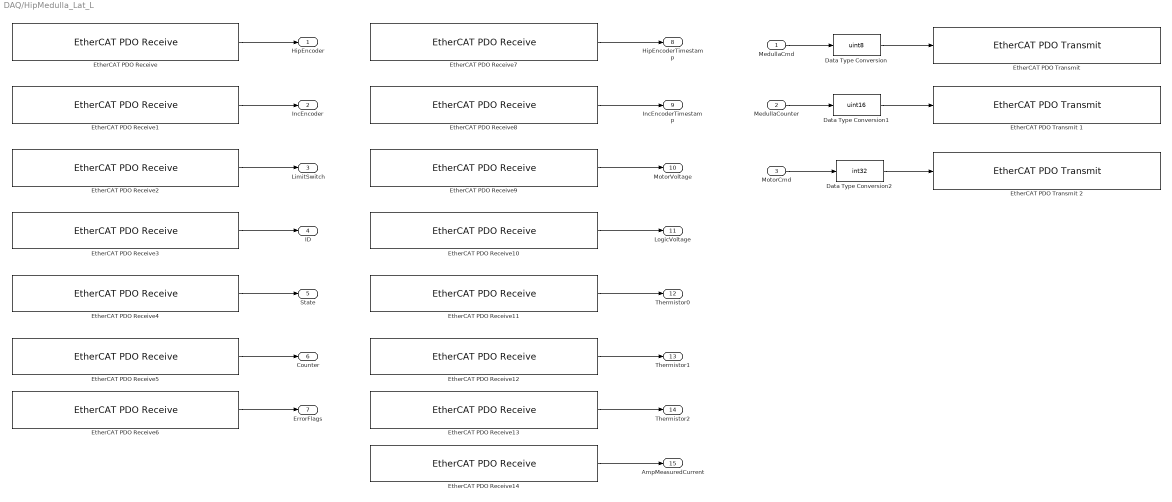
== system DAQ/HipMedulla_Lat_L ==
  MedullaCmd : Inport
  MedullaCounter : Inport  Port=2
  MotorCmd : Inport  Port=3
  Data Type Conversion : DataTypeConversion  OutDataTypeStr=uint8
  Data Type Conversion1 : DataTypeConversion  OutDataTypeStr=uint16
  Data Type Conversion2 : DataTypeConversion  OutDataTypeStr=int32
  EtherCAT PDO Receive : xpcethercatlib/EtherCAT PDO Receive  Priority=2  sig_name=Box 5 (ATRIAS 2.1 Hip (Medulla 1.5)).Hip Encoder.Encoder  sig_offset=2008  sig_type=uint32  type_size=32  sig_dim=1  device_id=0  sample_time=0.001000
  EtherCAT PDO Receive1 : xpcethercatlib/EtherCAT PDO Receive  Priority=2  sig_name=Box 5 (ATRIAS 2.1 Hip (Medulla 1.5)).Incremental Encoder.Incremental Encoder  sig_offset=2152  sig_type=uint16  type_size=16  sig_dim=1  device_id=0  sample_time=0.001000
  EtherCAT PDO Receive10 : xpcethercatlib/EtherCAT PDO Receive  Priority=2  sig_name=Box 5 (ATRIAS 2.1 Hip (Medulla 1.5)).Power.Logic Voltage  sig_offset=2072  sig_type=uint16  type_size=16  sig_dim=1  device_id=0  sample_time=0.001000
  EtherCAT PDO Receive11 : xpcethercatlib/EtherCAT PDO Receive  Priority=2  sig_name=Box 5 (ATRIAS 2.1 Hip (Medulla 1.5)).Thermistors.Thermistor 0  sig_offset=2088  sig_type=uint16  type_size=16  sig_dim=1  device_id=0  sample_time=0.001000
  EtherCAT PDO Receive12 : xpcethercatlib/EtherCAT PDO Receive  Priority=2  sig_name=Box 5 (ATRIAS 2.1 Hip (Medulla 1.5)).Thermistors.Thermistor 1  sig_offset=2104  sig_type=uint16  type_size=16  sig_dim=1  device_id=0  sample_time=0.001000
  EtherCAT PDO Receive13 : xpcethercatlib/EtherCAT PDO Receive  Priority=2  sig_name=Box 5 (ATRIAS 2.1 Hip (Medulla 1.5)).Thermistors.Thermistor 2  sig_offset=2120  sig_type=uint16  type_size=16  sig_dim=1  device_id=0  sample_time=0.001000
  EtherCAT PDO Receive14 : xpcethercatlib/EtherCAT PDO Receive  Priority=2  sig_name=Box 5 (ATRIAS 2.1 Hip (Medulla 1.5)).Measured Current.Amp Measured Current  sig_offset=2136  sig_type=int16  type_size=16  sig_dim=1  device_id=0  sample_time=0.001000
  EtherCAT PDO Receive2 : xpcethercatlib/EtherCAT PDO Receive  Priority=2  sig_name=Box 5 (ATRIAS 2.1 Hip (Medulla 1.5)).uController Status.Limit Switch  sig_offset=2000  sig_type=uint8  type_size=8  sig_dim=1  device_id=0  sample_time=0.001000
  EtherCAT PDO Receive3 : xpcethercatlib/EtherCAT PDO Receive  Priority=2  sig_name=Box 5 (ATRIAS 2.1 Hip (Medulla 1.5)).uController Status.ID  sig_offset=1968  sig_type=uint8  type_size=8  sig_dim=1  device_id=0  sample_time=0.001000
  EtherCAT PDO Receive4 : xpcethercatlib/EtherCAT PDO Receive  Priority=2  sig_name=Box 5 (ATRIAS 2.1 Hip (Medulla 1.5)).uController Status.State  sig_offset=1976  sig_type=uint8  type_size=8  sig_dim=1  device_id=0  sample_time=0.001000
  EtherCAT PDO Receive5 : xpcethercatlib/EtherCAT PDO Receive  Priority=2  sig_name=Box 5 (ATRIAS 2.1 Hip (Medulla 1.5)).uController Status.Counter  sig_offset=1984  sig_type=uint8  type_size=8  sig_dim=1  device_id=0  sample_time=0.001000
  EtherCAT PDO Receive6 : xpcethercatlib/EtherCAT PDO Receive  Priority=2  sig_name=Box 5 (ATRIAS 2.1 Hip (Medulla 1.5)).uController Status.Error Flags  sig_offset=1992  sig_type=uint8  type_size=8  sig_dim=1  device_id=0  sample_time=0.001000
  EtherCAT PDO Receive7 : xpcethercatlib/EtherCAT PDO Receive  Priority=2  sig_name=Box 5 (ATRIAS 2.1 Hip (Medulla 1.5)).Hip Encoder.Timestamp  sig_offset=2040  sig_type=uint16  type_size=16  sig_dim=1  device_id=0  sample_time=0.001000
  EtherCAT PDO Receive8 : xpcethercatlib/EtherCAT PDO Receive  Priority=2  sig_name=Box 5 (ATRIAS 2.1 Hip (Medulla 1.5)).Incremental Encoder.Incremental Encoder Timestamp  sig_offset=2168  sig_type=uint16  type_size=16  sig_dim=1  device_id=0  sample_time=0.001000
  EtherCAT PDO Receive9 : xpcethercatlib/EtherCAT PDO Receive  Priority=2  sig_name=Box 5 (ATRIAS 2.1 Hip (Medulla 1.5)).Power.Motor Voltage  sig_offset=2056  sig_type=uint16  type_size=16  sig_dim=1  device_id=0  sample_time=0.001000
  EtherCAT PDO Transmit : xpcethercatlib/EtherCAT PDO Transmit   Priority=3  sig_name=Box 5 (ATRIAS 2.1 Hip (Medulla 1.5)).uControllerInput.Command  sig_offset=1968  sig_type=uint8  type_size=8  sig_dim=1  device_id=0  sample_time=0.001000
  "EtherCAT PDO Transmit 1 " : xpcethercatlib/EtherCAT PDO Transmit   Priority=3  sig_name=Box 5 (ATRIAS 2.1 Hip (Medulla 1.5)).uControllerInput.Counter  sig_offset=1976  sig_type=uint16  type_size=16  sig_dim=1  device_id=0  sample_time=0.001000
  EtherCAT PDO Transmit 2 : xpcethercatlib/EtherCAT PDO Transmit   Priority=3  sig_name=Box 5 (ATRIAS 2.1 Hip (Medulla 1.5)).uControllerInput.Motor Current  sig_offset=1992  sig_type=int32  type_size=32  sig_dim=1  device_id=0  sample_time=0.001000
  HipEncoder : Outport
  IncEncoder : Outport  Port=2
  LimitSwitch : Outport  Port=3
  ID : Outport  Port=4
  State : Outport  Port=5
  Counter : Outport  Port=6
  ErrorFlags : Outport  Port=7
  HipEncoderTimestamp : Outport  Port=8
  IncEncoderTimestamp : Outport  Port=9
  MotorVoltage : Outport  Port=10
  LogicVoltage : Outport  Port=11
  Thermistor0 : Outport  Port=12
  Thermistor1 : Outport  Port=13
  Thermistor2 : Outport  Port=14
  AmpMeasuredCurrent : Outport  Port=15
  wires:
  Data Type Conversion/1 -> EtherCAT PDO Transmit/1
  Data Type Conversion1/1 -> "EtherCAT PDO Transmit 1 "/1
  Data Type Conversion2/1 -> EtherCAT PDO Transmit 2/1
  MedullaCmd/1 -> Data Type Conversion/1
  MedullaCounter/1 -> Data Type Conversion1/1
  MotorCmd/1 -> Data Type Conversion2/1
  EtherCAT PDO Receive8/1 -> IncEncoderTimestamp/1
  EtherCAT PDO Receive/1 -> HipEncoder/1
  EtherCAT PDO Receive7/1 -> HipEncoderTimestamp/1
  EtherCAT PDO Receive1/1 -> IncEncoder/1
  EtherCAT PDO Receive5/1 -> Counter/1
  EtherCAT PDO Receive3/1 -> ID/1
  EtherCAT PDO Receive2/1 -> LimitSwitch/1
  EtherCAT PDO Receive4/1 -> State/1
  EtherCAT PDO Receive6/1 -> ErrorFlags/1
  EtherCAT PDO Receive10/1 -> LogicVoltage/1
  EtherCAT PDO Receive9/1 -> MotorVoltage/1
  EtherCAT PDO Receive11/1 -> Thermistor0/1
  EtherCAT PDO Receive12/1 -> Thermistor1/1
  EtherCAT PDO Receive13/1 -> Thermistor2/1
  EtherCAT PDO Receive14/1 -> AmpMeasuredCurrent/1

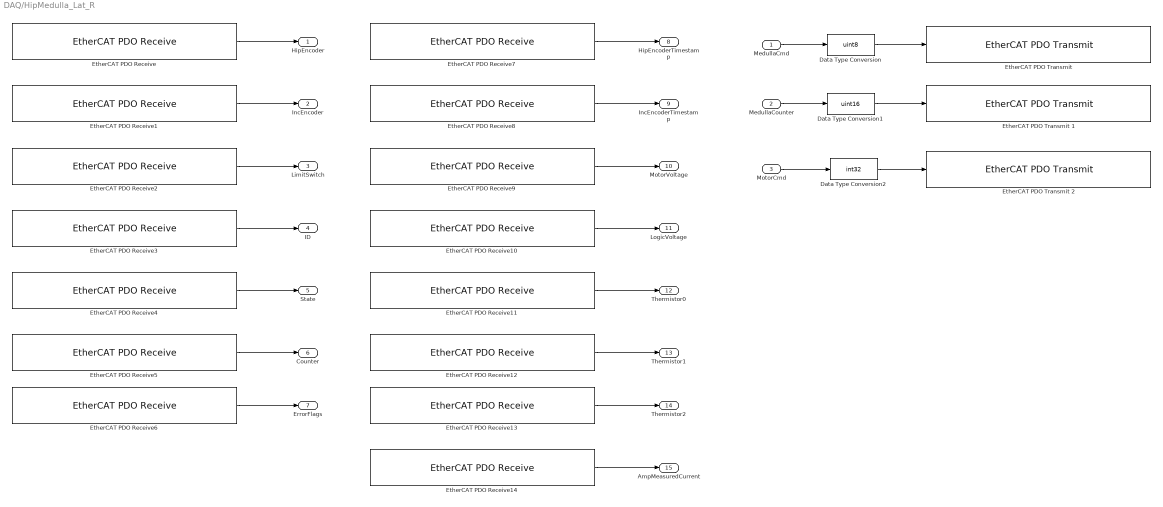
== system DAQ/HipMedulla_Lat_R ==
  MedullaCmd : Inport
  MedullaCounter : Inport  Port=2
  MotorCmd : Inport  Port=3
  Data Type Conversion : DataTypeConversion  OutDataTypeStr=uint8
  Data Type Conversion1 : DataTypeConversion  OutDataTypeStr=uint16
  Data Type Conversion2 : DataTypeConversion  OutDataTypeStr=int32
  EtherCAT PDO Receive : xpcethercatlib/EtherCAT PDO Receive  Priority=2  sig_name=Box 6 (ATRIAS 2.1 Hip (Medulla 1.5)).Hip Encoder.Encoder  sig_offset=2224  sig_type=uint32  type_size=32  sig_dim=1  device_id=0  sample_time=0.001000
  EtherCAT PDO Receive1 : xpcethercatlib/EtherCAT PDO Receive  Priority=2  sig_name=Box 6 (ATRIAS 2.1 Hip (Medulla 1.5)).Incremental Encoder.Incremental Encoder  sig_offset=2368  sig_type=uint16  type_size=16  sig_dim=1  device_id=0  sample_time=0.001000
  EtherCAT PDO Receive10 : xpcethercatlib/EtherCAT PDO Receive  Priority=2  sig_name=Box 6 (ATRIAS 2.1 Hip (Medulla 1.5)).Power.Logic Voltage  sig_offset=2288  sig_type=uint16  type_size=16  sig_dim=1  device_id=0  sample_time=0.001000
  EtherCAT PDO Receive11 : xpcethercatlib/EtherCAT PDO Receive  Priority=2  sig_name=Box 6 (ATRIAS 2.1 Hip (Medulla 1.5)).Thermistors.Thermistor 0  sig_offset=2304  sig_type=uint16  type_size=16  sig_dim=1  device_id=0  sample_time=0.001000
  EtherCAT PDO Receive12 : xpcethercatlib/EtherCAT PDO Receive  Priority=2  sig_name=Box 6 (ATRIAS 2.1 Hip (Medulla 1.5)).Thermistors.Thermistor 1  sig_offset=2320  sig_type=uint16  type_size=16  sig_dim=1  device_id=0  sample_time=0.001000
  EtherCAT PDO Receive13 : xpcethercatlib/EtherCAT PDO Receive  Priority=2  sig_name=Box 6 (ATRIAS 2.1 Hip (Medulla 1.5)).Thermistors.Thermistor 2  sig_offset=2336  sig_type=uint16  type_size=16  sig_dim=1  device_id=0  sample_time=0.001000
  EtherCAT PDO Receive14 : xpcethercatlib/EtherCAT PDO Receive  Priority=2  sig_name=Box 6 (ATRIAS 2.1 Hip (Medulla 1.5)).Measured Current.Amp Measured Current  sig_offset=2352  sig_type=int16  type_size=16  sig_dim=1  device_id=0  sample_time=0.001000
  EtherCAT PDO Receive2 : xpcethercatlib/EtherCAT PDO Receive  Priority=2  sig_name=Box 6 (ATRIAS 2.1 Hip (Medulla 1.5)).uController Status.Limit Switch  sig_offset=2216  sig_type=uint8  type_size=8  sig_dim=1  device_id=0  sample_time=0.001000
  EtherCAT PDO Receive3 : xpcethercatlib/EtherCAT PDO Receive  Priority=2  sig_name=Box 6 (ATRIAS 2.1 Hip (Medulla 1.5)).uController Status.ID  sig_offset=2184  sig_type=uint8  type_size=8  sig_dim=1  device_id=0  sample_time=0.001000
  EtherCAT PDO Receive4 : xpcethercatlib/EtherCAT PDO Receive  Priority=2  sig_name=Box 6 (ATRIAS 2.1 Hip (Medulla 1.5)).uController Status.State  sig_offset=2192  sig_type=uint8  type_size=8  sig_dim=1  device_id=0  sample_time=0.001000
  EtherCAT PDO Receive5 : xpcethercatlib/EtherCAT PDO Receive  Priority=2  sig_name=Box 6 (ATRIAS 2.1 Hip (Medulla 1.5)).uController Status.Counter  sig_offset=2200  sig_type=uint8  type_size=8  sig_dim=1  device_id=0  sample_time=0.001000
  EtherCAT PDO Receive6 : xpcethercatlib/EtherCAT PDO Receive  Priority=2  sig_name=Box 6 (ATRIAS 2.1 Hip (Medulla 1.5)).uController Status.Error Flags  sig_offset=2208  sig_type=uint8  type_size=8  sig_dim=1  device_id=0  sample_time=0.001000
  EtherCAT PDO Receive7 : xpcethercatlib/EtherCAT PDO Receive  Priority=2  sig_name=Box 6 (ATRIAS 2.1 Hip (Medulla 1.5)).Hip Encoder.Timestamp  sig_offset=2256  sig_type=uint16  type_size=16  sig_dim=1  device_id=0  sample_time=0.001000
  EtherCAT PDO Receive8 : xpcethercatlib/EtherCAT PDO Receive  Priority=2  sig_name=Box 6 (ATRIAS 2.1 Hip (Medulla 1.5)).Incremental Encoder.Incremental Encoder Timestamp  sig_offset=2384  sig_type=uint16  type_size=16  sig_dim=1  device_id=0  sample_time=0.001000
  EtherCAT PDO Receive9 : xpcethercatlib/EtherCAT PDO Receive  Priority=2  sig_name=Box 6 (ATRIAS 2.1 Hip (Medulla 1.5)).Power.Motor Voltage  sig_offset=2272  sig_type=uint16  type_size=16  sig_dim=1  device_id=0  sample_time=0.001000
  "EtherCAT PDO Transmit " : xpcethercatlib/EtherCAT PDO Transmit   Priority=3  sig_name=Box 6 (ATRIAS 2.1 Hip (Medulla 1.5)).uControllerInput.Command  sig_offset=2184  sig_type=uint8  type_size=8  sig_dim=1  device_id=0  sample_time=0.001000
  EtherCAT PDO Transmit 1 : xpcethercatlib/EtherCAT PDO Transmit   Priority=3  sig_name=Box 6 (ATRIAS 2.1 Hip (Medulla 1.5)).uControllerInput.Counter  sig_offset=2192  sig_type=uint16  type_size=16  sig_dim=1  device_id=0  sample_time=0.001000
  EtherCAT PDO Transmit 2 : xpcethercatlib/EtherCAT PDO Transmit   Priority=3  sig_name=Box 6 (ATRIAS 2.1 Hip (Medulla 1.5)).uControllerInput.Motor Current  sig_offset=2208  sig_type=int32  type_size=32  sig_dim=1  device_id=0  sample_time=0.001000
  HipEncoder : Outport
  IncEncoder : Outport  Port=2
  LimitSwitch : Outport  Port=3
  ID : Outport  Port=4
  State : Outport  Port=5
  Counter : Outport  Port=6
  ErrorFlags : Outport  Port=7
  HipEncoderTimestamp : Outport  Port=8
  IncEncoderTimestamp : Outport  Port=9
  MotorVoltage : Outport  Port=10
  LogicVoltage : Outport  Port=11
  Thermistor0 : Outport  Port=12
  Thermistor1 : Outport  Port=13
  Thermistor2 : Outport  Port=14
  AmpMeasuredCurrent : Outport  Port=15
  wires:
  Data Type Conversion/1 -> "EtherCAT PDO Transmit "/1
  Data Type Conversion1/1 -> EtherCAT PDO Transmit 1/1
  Data Type Conversion2/1 -> EtherCAT PDO Transmit 2/1
  MedullaCmd/1 -> Data Type Conversion/1
  MedullaCounter/1 -> Data Type Conversion1/1
  MotorCmd/1 -> Data Type Conversion2/1
  EtherCAT PDO Receive8/1 -> IncEncoderTimestamp/1
  EtherCAT PDO Receive/1 -> HipEncoder/1
  EtherCAT PDO Receive7/1 -> HipEncoderTimestamp/1
  EtherCAT PDO Receive1/1 -> IncEncoder/1
  EtherCAT PDO Receive5/1 -> Counter/1
  EtherCAT PDO Receive3/1 -> ID/1
  EtherCAT PDO Receive2/1 -> LimitSwitch/1
  EtherCAT PDO Receive4/1 -> State/1
  EtherCAT PDO Receive6/1 -> ErrorFlags/1
  EtherCAT PDO Receive10/1 -> LogicVoltage/1
  EtherCAT PDO Receive9/1 -> MotorVoltage/1
  EtherCAT PDO Receive11/1 -> Thermistor0/1
  EtherCAT PDO Receive12/1 -> Thermistor1/1
  EtherCAT PDO Receive13/1 -> Thermistor2/1
  EtherCAT PDO Receive14/1 -> AmpMeasuredCurrent/1
